simulink model "FOPID_control_heat_pump"  (R2016a)
settings: Solver=ode23s  StartTime=0.0  StopTime=50  RelTol=1e-3
libraries: fod x1, fuzblock x1
settings Model: Creator=EBUKA  LastModifiedBy=EBUKA

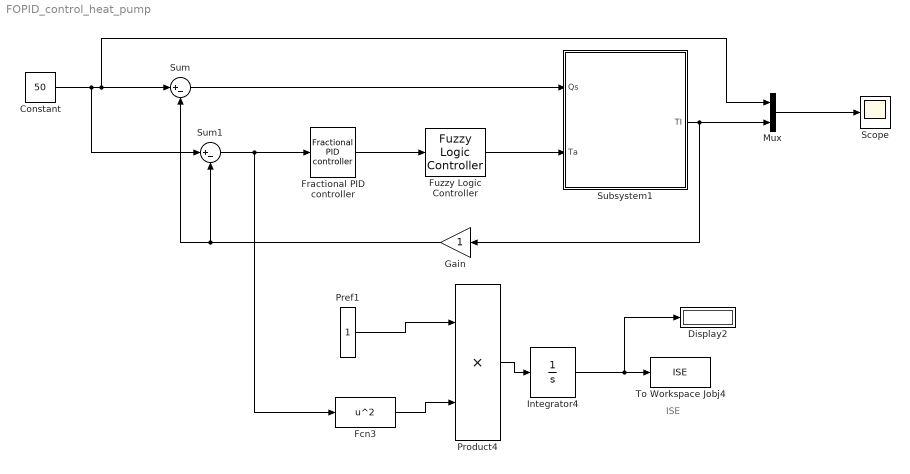
== system FOPID_control_heat_pump ==
  note: ISE
  Constant : Constant  Value=50
  Display2 : Display
  Fcn3 : Fcn  Expr=u^2
  Fractional PID controller : fod/Fractional PID controller  Kp=0.2544  Ki=1  lambda=0.4635  Kd=0.9604  mic=0.2875  freqRange=[0.001, 1000]  N=5
  Fuzzy Logic Controller : fuzblock/Fuzzy Logic  Controller  fis=Temp
  Gain : Gain
  Integrator4 : Integrator
  Mux : Mux  Inputs=2
  Pref1 : Constant
  Product4 : Product
  Scope : Scope
  Subsystem1 : Subsystem
  Sum : Sum  Inputs=|+-
  Sum1 : Sum  Inputs=|+-
  To Workspace Jobj4 : ToWorkspace  VariableName=ISE  SampleTime=-1
  wires:
  Constant/1 -> Sum1/1, Mux/1, Sum/1
  Subsystem1/1(TI) -> Gain/1, Mux/2
  Sum/1 -> Subsystem1/1(Qs)
  Gain/1 -> Sum1/2, Sum/2
  Mux/1 -> Scope/1
  Fractional PID controller/1 -> Fuzzy Logic Controller/1
  Product4/1 -> Integrator4/1
  Integrator4/1 -> To Workspace Jobj4/1, Display2/1
  Fcn3/1 -> Product4/2
  Pref1/1 -> Product4/1
  Sum1/1 -> Fcn3/1, Fractional PID controller/1
  Fuzzy Logic Controller/1 -> Subsystem1/2(Ta)

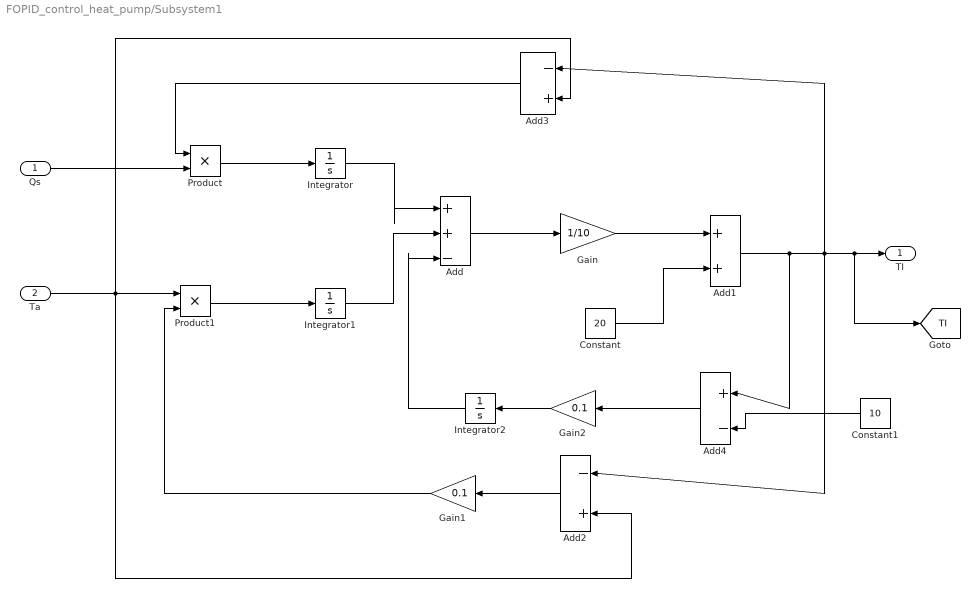
== system FOPID_control_heat_pump/Subsystem1 ==
  Qs : Inport
  Ta : Inport  Port=2
  Add : Sum  Inputs=|++-
  Add1 : Sum
  Add2 : Sum  Inputs=|-+
  Add3 : Sum  Inputs=|-+
  Add4 : Sum  Inputs=|+-
  Constant : Constant  Value=20
  Constant1 : Constant  Value=10
  Gain : Gain  Gain=1/10
  Gain1 : Gain  Gain=0.1
  Gain2 : Gain  Gain=0.1
  Integrator : Integrator
  Integrator1 : Integrator
  Integrator2 : Integrator
  Product : Product
  Product1 : Product
  TI : Outport
  tag scope: TI=global
  wires:
  Add2/1 -> Gain1/1
  Gain1/1 -> Product1/2
  Qs/1 -> Product/2
  Integrator1/1 -> Add/2
  Product/1 -> Integrator/1
  Add/1 -> Gain/1
  Constant1/1 -> Add4/2
  Add4/1 -> Gain2/1
  Gain/1 -> Add1/1
  Gain2/1 -> Integrator2/1
  Integrator2/1 -> Add/3
  Ta/1 -> Add3/2, Add2/2, Product1/1
  Constant/1 -> Add1/2
  Add1/1 -> Add4/1, [TI], TI/1, Add3/1, Add2/1
  Integrator/1 -> Add/1
  Product1/1 -> Integrator1/1
  Add3/1 -> Product/1
